simulink model "hw5"  (R2017a)
settings: Solver=VariableStepAuto  StartTime=0.0  StopTime=10.0  RelTol=1e-3
libraries: dspsrcs4 x1
settings Model: Creator=Jessica  LastModifiedBy=Jessica

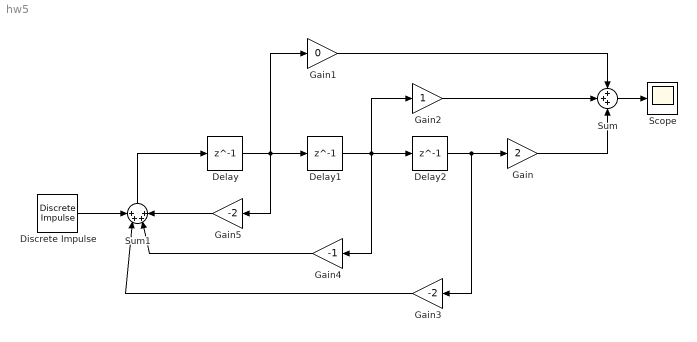
== system hw5 ==
  Delay : Delay  DelayLength=1  InitialCondition=0
  Delay1 : Delay  DelayLength=1  InitialCondition=0
  Delay2 : Delay  DelayLength=1  InitialCondition=0
  Discrete Impulse : dspsrcs4/Discrete  Impulse  Delay=0  SampleTime=1  FrameSample=1  OutputFrames=off  dataType=double  isSigned=on  wordLen=16  udDataType=sfix(16)  fracBitsMode=Best precision  numFracBits=15  OutDataTypeStr=double  LastOutDataTypeStr=double
  Gain : Gain  Gain=2
  Gain1 : Gain  Gain=0
  Gain2 : Gain
  Gain3 : Gain  Gain=-2
  Gain4 : Gain  Gain=-1
  Gain5 : Gain  Gain=-2
  Scope : Scope
  Sum : Sum  Inputs=+++
  Sum1 : Sum  Inputs=++++
  wires:
  Delay2/1 -> Gain3/1, Gain/1
  Sum1/1 -> Delay/1
  Gain/1 -> Sum/3
  Gain2/1 -> Sum/2
  Gain1/1 -> Sum/1
  Gain5/1 -> Sum1/4
  Gain4/1 -> Sum1/3
  Gain3/1 -> Sum1/2
  Delay/1 -> Gain5/1, Gain1/1, Delay1/1
  Delay1/1 -> Gain4/1, Gain2/1, Delay2/1
  Discrete Impulse/1 -> Sum1/1
  Sum/1 -> Scope/1
